simulink model "Homework_ch12"  (R2021b)
settings: Solver=VariableStepAuto  StartTime=0.0  StopTime=10.0  RelTol=1e-3
settings Model: Creator=86195  LastModifiedBy=86195

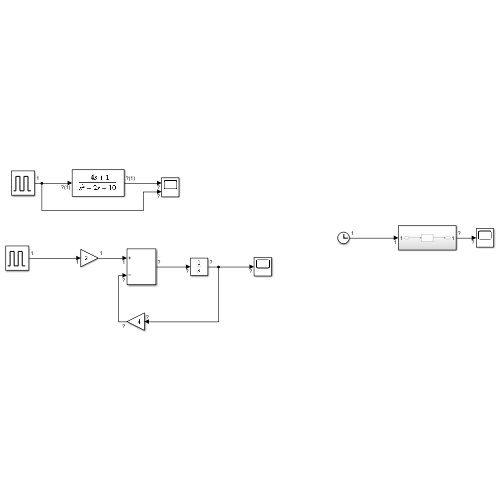
[thumbnail: Simulink's stored preview of the top-level diagram]
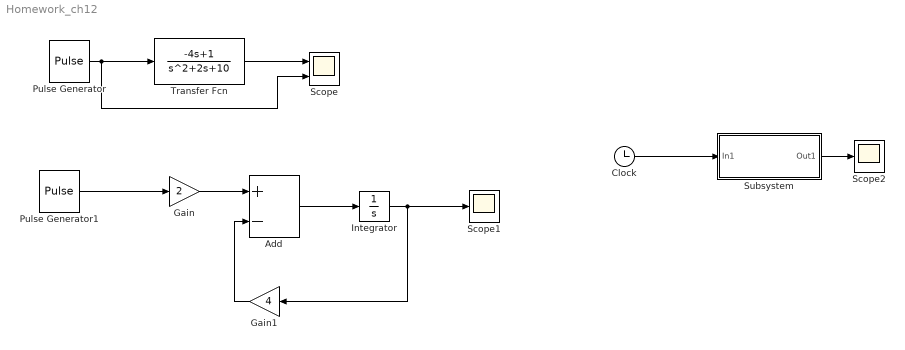
== system Homework_ch12 ==
  Add : Sum  Inputs=+-
  Clock : Clock
  Gain : Gain  Gain=2
  Gain1 : Gain  Gain=4
  Integrator : Integrator
  Pulse Generator : DiscretePulseGenerator  PulseType=Time based  Period=10  PulseWidth=5
  Pulse Generator1 : DiscretePulseGenerator  PulseType=Time based  Period=1  PulseWidth=50
  Scope : Scope  NumInputPorts=2
  Scope1 : Scope
  Scope2 : Scope
  Subsystem : Subsystem
  Transfer Fcn : TransferFcn  Numerator=[-4 1]  Denominator=[1 2 10]
  wires:
  Pulse Generator/1 -> Scope/2, Transfer Fcn/1
  Transfer Fcn/1 -> Scope/1
  Pulse Generator1/1 -> Gain/1
  Gain/1 -> Add/1
  Add/1 -> Integrator/1
  Integrator/1 -> Gain1/1, Scope1/1
  Gain1/1 -> Add/2
  Clock/1 -> Subsystem/1(In1)
  Subsystem/1(Out1) -> Scope2/1

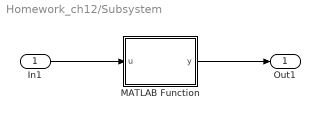
== system Homework_ch12/Subsystem ==
  In1 : Inport
  MATLAB Function : MATLAB Function  TreatAsAtomicUnit=on
  Out1 : Outport
  wires:
  In1/1 -> MATLAB Function/1(u)
  MATLAB Function/1(y) -> Out1/1

== matlab function Homework_ch12/Subsystem/MATLAB Function ==
  data: u input; y output
function y = fcn(u)

y = 2*exp(-0.5*x)*sin(2*pi*x);
